simulink model "closedloop_speed_controller"  (R2023b)
settings: Solver=VariableStepAuto  StartTime=0.0  StopTime=10.0  RelTol=1e-3
libraries: spsSeriesRLCBranchLib x2, spsCurrentMeasurementLib x1, spsDCMachineLib x1, spsDCVoltageSourceLib x1, spsDiodeLib x1, spsIdealSwitchLib x1, simulink x1, spspowerguiLib x1
settings Model: Creator=sraya  LastModifiedBy=sraya

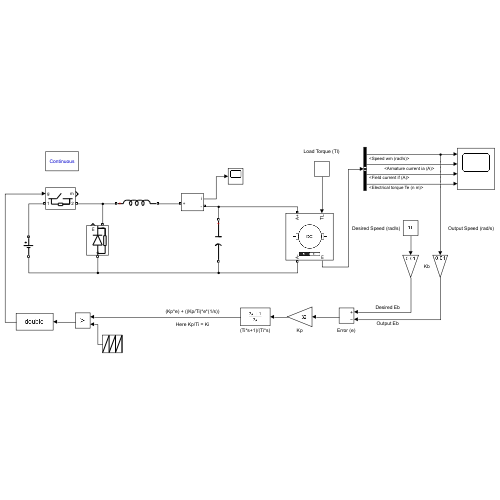
[thumbnail: Simulink's stored preview of the top-level diagram]
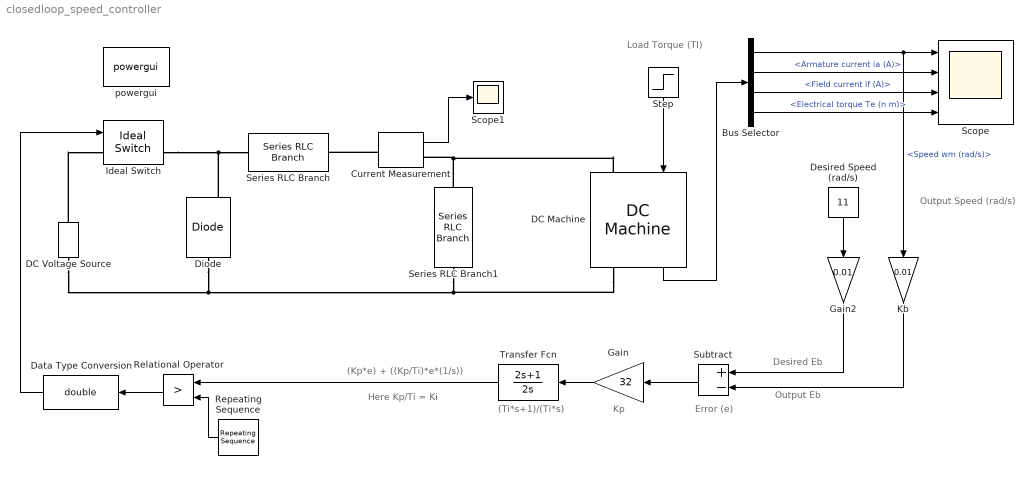
== system closedloop_speed_controller ==
  note: Load Torque (Tl)
  note: Output Speed (rad/s)
  note: Output Eb
  note: Kp
  note: Here Kp/Ti = Ki
  note: (Ti*s+1)/(Ti*s)
  note: Desired Eb
  note: (Kp*e) + ((Kp/Ti)*e*(1/s))
  note: Error (e)
  Bus Selector : BusSelector  OutputSignals=Speed wm (rad/s),Armature current ia (A),Field current if (A),Electrical torque Te (n m)
  Current Measurement : spsCurrentMeasurementLib/Current Measurement  PhasorSimulation=off  OutputType=Complex  PSBequivalent=0
  DC Machine : spsDCMachineLib/DC Machine  PresetModel=No  MechanicalLoad=Torque TL  FieldType=Permanent magnet  ShowDetailedParameters=on  MeasurementBus=off  RLa="[ 1  0.5]"  RLf="[ 240  120]"  Laf=1.8  MachineConstant=Torque constant (N.m/A)  Ke=0.01  Kt=0.01  J=0.01  Bm=0.1  Tf=0  w0=0  Ifinit=0  TsPowergui=0  TsBlock=-1
  DC Voltage Source : spsDCVoltageSourceLib/DC Voltage Source  Amplitude=220  Measurements=Voltage
  Data Type Conversion : DataTypeConversion  OutDataTypeStr=double  SaturateOnIntegerOverflow=off  RndMeth=Floor
  Desired Speed (rad/s) : Constant  Value=11
  Diode : spsDiodeLib/Diode  Ron=0.001  Lon=0  Vf=0.8  IC=0  UseSnubber=off  Rs=500  Cs=250e-9  Measurements=on
  Gain : Gain  Gain=32
  Gain2 : Gain  Gain=0.01
  Ideal Switch : spsIdealSwitchLib/Ideal Switch  Ron=0.001  Lon=0  IC=0  Rs=1e5  Cs=inf  Measurements=on
  Kb : Gain  Gain=0.01
  Relational Operator : RelationalOperator  Operator=>  OutDataTypeStr=boolean  InputSameDT=off
  Repeating Sequence : simulink/Sources/Repeating Sequence  rep_seq_t=[0 0.0002]  rep_seq_y=[0 1]
  Scope : Scope  NumInputPorts=4
  Scope1 : Scope
  Series RLC Branch : spsSeriesRLCBranchLib/Series RLC Branch  LConnTagsString=__new0  RConnTagsString=__new0  BranchType=L  Resistance=1  Inductance=0.1  SetiL0=off  InitialCurrent=0  Capacitance=1e-6  Setx0=off  InitialVoltage=0  Measurements=None
  Series RLC Branch1 : spsSeriesRLCBranchLib/Series RLC Branch  LConnTagsString=__new0  RConnTagsString=__new0  BranchType=C  Resistance=1  Inductance=1e-3  SetiL0=off  InitialCurrent=0  Capacitance=5e-6  Setx0=off  InitialVoltage=0  Measurements=None
  Step : Step  Time=0.55  After=0.8  SampleTime=0
  Subtract : Sum  Inputs=+-
  Transfer Fcn : TransferFcn  Numerator=[2 1]  Denominator=[2 0]
  powergui : spspowerguiLib/powergui  Priority=1  SimulationMode=Continuous  SampleTime=50e-6  frequency=60  Iterations=50  frequencyindice=0  Pbase=100e6  ErrMax=1e-4  UnitsV=kV  UnitsW=MW  buscounter=0  FunctionMessages=off  echomessages=off  EnableUseOfTLC=off  CurrentSourceSwitches=off  DisableSnubberDevices=off  DisableRonSwitches=off  DisableVfSwitches=off  DisplayEquations=off  AutomaticDiscreteSolvers=off  SolverType=Tustin/Backward Euler (TBE)  Interpol=off  ExternalGateDelay=off  methode=off  Ts=10  x0status=blocks  SPID=on  SwTol=0  HookPort=off  NonlinearTolerance=1e-4  nMaxIteration=100  ContinueOnMaxIteration=off  RestoreLinks=warning  ResistiveCurrentMeasurement=off  Frange=[0:2:500]  Ylog=off  Xlog=on  ShowGrid=off  save=off  variable=ZData  structure=0  ZoomFFT=off  StartTime=0.0  cycles=1  DisplayStyle=1  fundamental=60  FreqAxis=off  MaxFrequency=1000  frequencyindicesteady=1  RmsSteady=1  display=off
  wires:
  Bus Selector/2 -> Scope/2  "<Armature current ia (A)>"
  Bus Selector/4 -> Scope/4  "<Electrical torque Te (n m)>"
  Kb/1 -> Subtract/2
  Gain2/1 -> Subtract/1
  Step/1 -> DC Machine/1
  Bus Selector/3 -> Scope/3  "<Field current if (A)>"
  Current Measurement/1 -> Scope1/1
  Gain/1 -> Transfer Fcn/1
  Subtract/1 -> Gain/1
  Bus Selector/1 -> Scope/1, Kb/1  "<Speed wm (rad/s)>"
  Repeating Sequence/1 -> Relational Operator/2
  Transfer Fcn/1 -> Relational Operator/1
  Data Type Conversion/1 -> Ideal Switch/1
  Relational Operator/1 -> Data Type Conversion/1
  Desired Speed (rad/s)/1 -> Gain2/1
  DC Machine/1 -> Bus Selector/1
  connections:
  DC Machine/LConn1 -- Series RLC Branch1/LConn1 -- Current Measurement/RConn1
  Diode/RConn1 -- Series RLC Branch/LConn1 -- Ideal Switch/RConn1
  Diode/LConn1 -- DC Voltage Source/LConn1 -- Series RLC Branch1/RConn1 -- DC Machine/RConn1
  DC Voltage Source/RConn1 -- Ideal Switch/LConn1
  Current Measurement/LConn1 -- Series RLC Branch/RConn1
